simulink model "consolidate_sensors"  (R2025b)
settings: Solver=VariableStepAuto  StartTime=0.0  StopTime=10.0  RelTol=1e-3
settings Model: Creator=atcushen  LastModifiedBy=atcushen

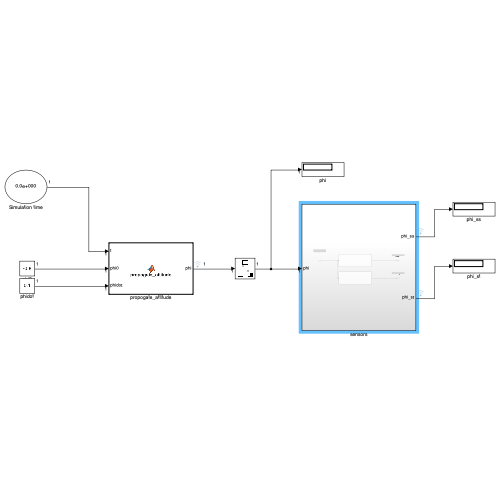
[thumbnail: Simulink's stored preview of the top-level diagram]
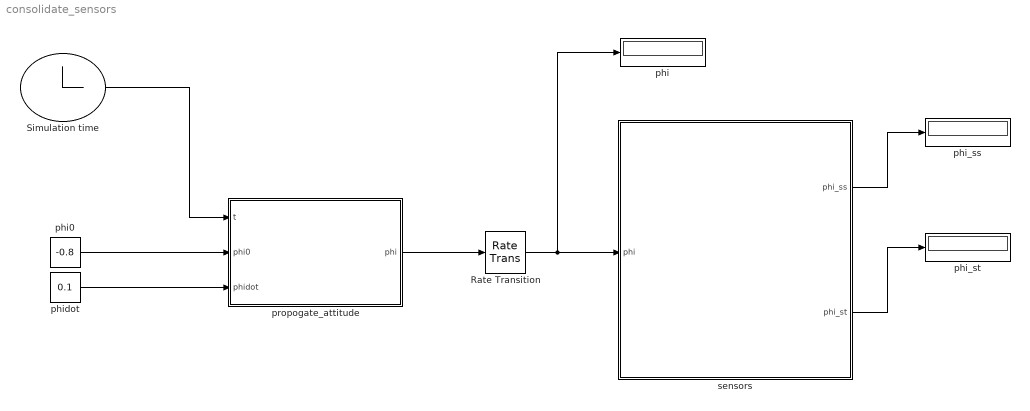
== system consolidate_sensors ==
  Rate Transition : RateTransition  OutPortSampleTime=0.5
  Simulation time : Clock
  phi : Display
  phi0 : Constant  Value=-0.8
  phi_ss : Display
  phi_st : Display
  phidot : Constant  Value=0.1
  propogate_attitude : MATLAB Function  TreatAsAtomicUnit=on
  sensors : Subsystem
  wires:
  sensors/2(phi_st) -> phi_st/1
  Rate Transition/1 -> phi/1, sensors/1(phi)
  phidot/1 -> propogate_attitude/3(phidot)
  Simulation time/1 -> propogate_attitude/1(t)
  phi0/1 -> propogate_attitude/2(phi0)
  sensors/1(phi_ss) -> phi_ss/1
  propogate_attitude/1(phi) -> Rate Transition/1

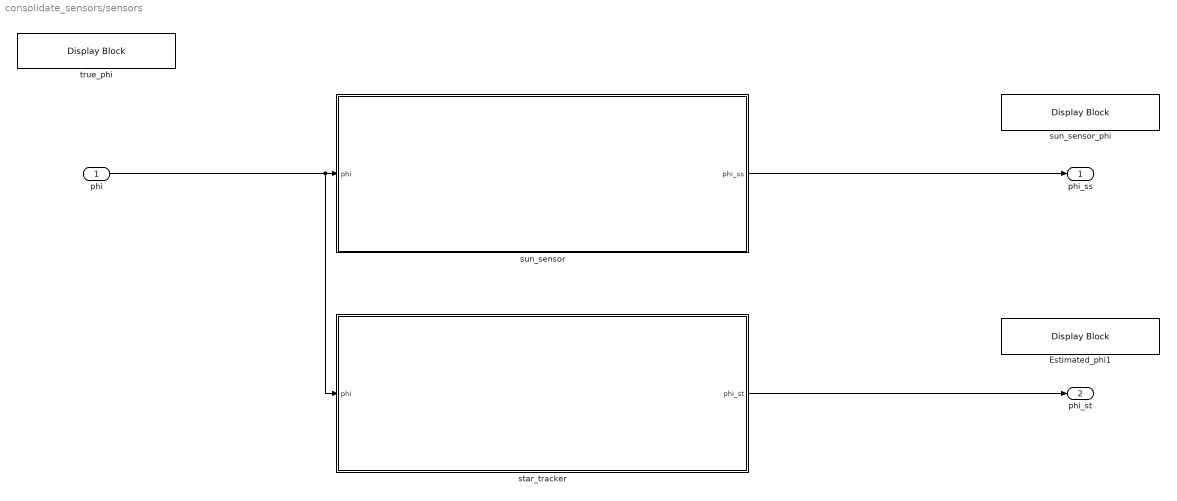
== system consolidate_sensors/sensors ==
  phi : Inport
  Estimated_phi1 : DisplayBlock  LabelPosition=Bottom  Transparency=1  GridColor=[0.502, 0.502, 0.502]
  star_tracker : Subsystem
  sun_sensor : Subsystem
  sun_sensor_phi : DisplayBlock  LabelPosition=Bottom  Transparency=1  GridColor=[0.502, 0.502, 0.502]
  true_phi : DisplayBlock  LabelPosition=Hide  Transparency=1  GridColor=[0.502, 0.502, 0.502]
  phi_ss : Outport
  phi_st : Outport  Port=2
  wires:
  phi/1 -> star_tracker/1(phi), sun_sensor/1(phi)
  sun_sensor/1(phi_ss) -> phi_ss/1
  star_tracker/1(phi_st) -> phi_st/1

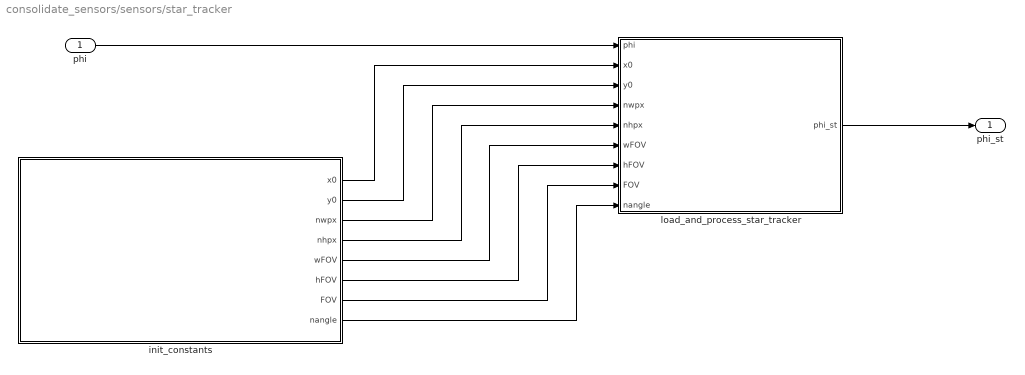
== system consolidate_sensors/sensors/star_tracker ==
  phi : Inport
  init_constants : MATLAB Function  TreatAsAtomicUnit=on
  load_and_process_star_tracker : MATLAB Function  TreatAsAtomicUnit=on
  phi_st : Outport
  wires:
  load_and_process_star_tracker/1(phi_st) -> phi_st/1
  init_constants/1(x0) -> load_and_process_star_tracker/2(x0)
  phi/1 -> load_and_process_star_tracker/1(phi)
  init_constants/2(y0) -> load_and_process_star_tracker/3(y0)
  init_constants/3(nwpx) -> load_and_process_star_tracker/4(nwpx)
  init_constants/4(nhpx) -> load_and_process_star_tracker/5(nhpx)
  init_constants/5(wFOV) -> load_and_process_star_tracker/6(wFOV)
  init_constants/6(hFOV) -> load_and_process_star_tracker/7(hFOV)
  init_constants/7(FOV) -> load_and_process_star_tracker/8(FOV)
  init_constants/8(nangle) -> load_and_process_star_tracker/9(nangle)

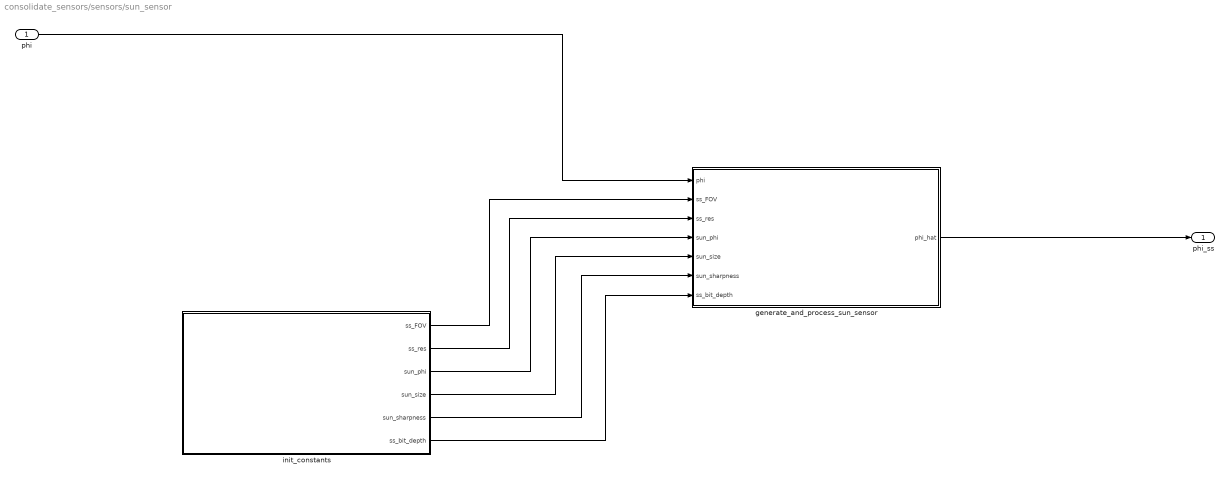
== system consolidate_sensors/sensors/sun_sensor ==
  phi : Inport
  generate_and_process_sun_sensor : MATLAB Function  TreatAsAtomicUnit=on
  init_constants : MATLAB Function  TreatAsAtomicUnit=on
  phi_ss : Outport
  wires:
  phi/1 -> generate_and_process_sun_sensor/1(phi)
  init_constants/5(sun_sharpness) -> generate_and_process_sun_sensor/6(sun_sharpness)
  init_constants/1(ss_FOV) -> generate_and_process_sun_sensor/2(ss_FOV)
  init_constants/2(ss_res) -> generate_and_process_sun_sensor/3(ss_res)
  init_constants/4(sun_size) -> generate_and_process_sun_sensor/5(sun_size)
  init_constants/3(sun_phi) -> generate_and_process_sun_sensor/4(sun_phi)
  init_constants/6(ss_bit_depth) -> generate_and_process_sun_sensor/7(ss_bit_depth)
  generate_and_process_sun_sensor/1(phi_hat) -> phi_ss/1

== matlab function consolidate_sensors/propogate_attitude ==
  data: t input; phi output; phi0 input; phidot input
% propogate attitude
function phi = propogate_attitude(t,phi0,phidot)
    % Input: 
    % t: float, current time, in s
    % phi0: float, initial attitude, in radians
    % phidot: float, rotation rate, in rad/sec
    
    % Output:
    % phi: float, current attitude, in rad/sec

    phi = mod(t*phidot + phi0 + pi,2*pi) - pi;
end

== matlab function consolidate_sensors/sensors/star_tracker/load_and_process_star_tracker ==
  data: phi_st output; phi input; x0 input; y0 input; nwpx input; nhpx input; wFOV input; hFOV input; FOV input; nangle input
function phi_st  = load_and_process_star_tracker(phi,x0,y0,nwpx,nhpx,wFOV,hFOV,FOV,nangle)
    
    % DEFINE PATHS TO STARFIELD IMAGE AND STARTABLE
    starfield_path = 'star_field2.mat'; % str, name of reference photo of full starfield image (which nwpx,wFOV etc describe)
    startable_path = 'star_table2.mat'; % str, name of table which identifies star locations, in radians 


    % PART 1: LOAD STAR TABLE
    
    struct = load(startable_path);
    star_table = struct.star_table;


    % PART 2: GENERATE LOOKUP TABLE

    % Input
    % star_table: nx3 array, from generate_star_table
    % nangle: integer, how many stars to compute angles to from reference
    % star

    % Output
    % star_lookup: nxnagle array, each row corresponds to given row in
    % star_table, columns are angular distances to nangle closest stars

    % Initialize lookup table
    star_lookup = zeros(size(star_table, 1), nangle);

    % Iterate through each star in the table
    for istar = 1:length(star_table)
        
        % Compute the angular distances from the current star to all other stars
        phi_diff = star_table(istar, 1) - star_table(:, 1);
        theta_diff = star_table(istar, 2) - star_table(:, 2);
        angle_diff = sqrt(phi_diff.^2 + theta_diff.^2);

        % Sort the angular distances and get the indices of the smallest values
        [sorted_angles, ~] = sort(angle_diff);
        star_lookup(istar, :) = sorted_angles(2:min(nangle+1, length(sorted_angles))); % Store the smallest values

    
    % PART 3: LOAD STARFIELD REFERENCE IMAGE, AND CROP TO DESIRED FOV

    % Input
    % image: str, path to .png field to import of starfield
    % phi: float, boresight angle of camera, in radians, from -pi to pi
    % FOV: float, angular field of view of camera, in radians, from 0 to 2pi
    % x0: int, x pixel coord of reference star 
    % y0: int, x pixel coord of reference star 
    % nwpx: int, number of pixels of width of starfield image
    % nhpx: int, number of pixels of height of starfield image
    % wFOV: float, field of view width of starfield image [deg]
    % hFOV: float, field of view height of starfield image [deg]
    % Output:
    % st_im: nres x nres array, representing synethic star tracker image

    % Load the .png image as a black and white image array
    file = load(starfield_path);
    img = file.img; 
    starfield_im = rgb2gray(img); % Convert the image to grayscale
    starfield_im = flip(starfield_im,1); % Image array is upside down)

    % Create coordinate axes
    x_ax = 1:nwpx - x0;
    y_ax = 1:nhpx - y0;
    phi_ax = x_ax * pi/180 * wFOV/nwpx;
    theta_ax = y_ax * pi/180 * hFOV/nhpx;
    
    % Crop the starfield image based on the field of view and the phi axis
    phi_indices = phi_ax >= (phi - FOV/2) & phi_ax <= (phi + FOV/2);
    theta_indices = theta_ax >= (-FOV/2) & theta_ax <= (FOV/2); %y0-round(nres/2):y0-round(nres/2)+nres-1;
    
    % Crop the image
    st_im = starfield_im(theta_indices, phi_indices);


    % PART 4: IDENTIFY STAR PIXEL CLUSTERS IN IMAGE

      % Input:
    % st_im: nxn array, representing image from star tracker
    % FOV: float, field of view along each edge of image
    % Output:
    % star_ls: nx2 array, the phi and theta positions (relative to the
    % center of the image) for each star identified
    
    % Get image dimensions (not passed to function call)
    [theta_nres,phi_nres] = size(st_im);
    
    % Convert coordinates to phi and theta positions
    phi_positions = linspace(-FOV/2, FOV/2, phi_nres);
    theta_positions = linspace(-FOV/2, FOV/2, theta_nres);
    
    % Identify bright points in the star tracker image
     threshold = 0.3 * 255; % Set a threshold to identify bright points
    % Create filtered im
     filtered_im = zeros(size(st_im)); % Initialize filtered image
     filtered_im(st_im > threshold) = 1; % Set values to 1 where st_im exceeds threshold
    % Find connected components
     CC = bwconncomp(filtered_im);
    % Create label matrix - CHANGED FOR CODEGEN
     L = zeros(size(filtered_im), 'uint16');
     for k = 1:CC.NumObjects
         L(CC.PixelIdxList{k}) = k;
     end
    % Create output array for star positions
     star_ls = zeros(max(L(:)), 2);
    % Iterate through each connected component
    for jstar = 1:max(L(:))
    % Get the coordinates of the current star cluster
     [y_cluster, x_cluster] = find(L == jstar);
    % Store the average position of the cluster
     star_ls(jstar, 1) = mean(phi_positions(x_cluster)); % Average phi coordinate
     star_ls(jstar, 2) = mean(theta_positions(y_cluster)); % Average theta coordinate
    end

    % PART 5: MATCH IDENTIFIED STARS TO LOOKUP TABLE

    % Input
    % star_ls: nx2 array, the phi and theta positions (relative to the
    % center of the image) for each star identified
    % star_pos_error: float, angular uncertainty in position of stars
    % star_lookup: nxnagle array, each row corresponds to given row in
    % star_table, columns are angular distances to closest stars

    % Output
    % star_num: integer, index number of matched star
    % deltaphi: float, offset in phi of matched star from image center, in radians
    % deltatheta: float, offset in phi of matched star from image center, in radians
    % match_status: integer, 0=failed, 1=matched, 2=multiple matches refined
    % stars_tried: integer, number of stars checked before finding match

    % Compute error bound as single pixel width (radians)
    star_pos_error = wFOV/nwpx * pi/180;

    % CHANGED FOR CODEGEN - Initialize outputs with default values
    star_num = int32(-1);
    deltaphi = 0.0;
    deltatheta = 0.0;
    match_status = int32(0);  % debug output
    stars_tried = int32(0);   % debug output

    % Iterate through stars in image, starting closest to middle, until we
    % get a positive match
    star_match = false;
    
    % Calculate the sum of squares for each star position
    star_ls_dist = sum(star_ls.^2, 2);
    
    % Sort the star_ls based on the sum of squares
    [~, sorted_indices] = sort(star_ls_dist);
    star_ls = star_ls(sorted_indices, :);

    istar = 1;
    while star_match == false && istar <= length(star_ls)
        stars_tried = int32(istar);  % tracking progress
        
        % Compute distances to other stars
        phi_diff = star_ls(istar, 1) - star_ls(:, 1);
        theta_diff = star_ls(istar, 2) - star_ls(:, 2);
        angle_diff = sqrt(phi_diff.^2 + theta_diff.^2);

        % Sort the computed angular distances from smallest to largest
        [sorted_angles, ~] = sort(angle_diff);
        
        % Drop the first element of sorted_angles (distance to itself = 0)
        sorted_angles(1) = [];

        % Reduce sorted angles to only be as long as star_lookup is wide
        sorted_angles = sorted_angles(1:min(length(sorted_angles), size(star_lookup, 2)));

        % Create an array of stars within the positional error range
        match_indices = star_lookup(:, 1) >= (sorted_angles(1) - star_pos_error) & ...
                        star_lookup(:, 1) <= (sorted_angles(1) + star_pos_error);
        matched_stars = star_lookup(match_indices, :);

        % Check if that immediately identified the current state. 
        % If not, compare the angular distances one by one, bringing in more to
        % reduce the number of remaining options
        iangle = 2;

        while size(matched_stars,1) > 1 & iangle <= size(star_lookup,2)
            match_status = int32(2);  % indicates multiple matches being refined
            
            % We loop through the remaining matches
            for j = 1:size(match_indices, 1)
                if j ~= 0
                    % Check to see if the next closest star is within error of
                    % any of the neighbouring stars listed in the lookup table
                    % If none of the angles are close enough, then reject this
                    % match
                    if all(abs(star_lookup(j, iangle:end) - sorted_angles(iangle)) > star_pos_error)
                        match_indices(j) = 0; % Set the jth non-zero element of match_indices to zero
                    end
                end 
            end
            matched_stars = star_lookup(match_indices, :);
        
            iangle = iangle + 1;
        end
        
        % Check if we could use this star 
        if size(matched_stars,1) ~= 1
            % no match found for this star, continue
            istar = istar + 1; % Move to the next star
        else
            % CHANGED FOR CODEGEN - Force scalar by using loop instead of find
            for k = 1:length(match_indices)
                if match_indices(k) ~= 0
                    star_num = int32(k);
                    break;
                end
            end
            deltaphi = star_ls(istar,1); % Offset in phi
            deltatheta = star_ls(istar,2); % Offset in theta
            star_match = true;
            match_status = int32(1);  % successful match
        end
    end

    % Return error if star tracker failed 
    if star_match == false
        % CHANGED FOR CODEGEN - tracker failed
        star_num = int32(-1);
        deltaphi = 0.0;
        deltatheta = 0.0;
        match_status = int32(0);  % Failed to match
    end

    
    % PART 6: COMPUTE PHI_HAT

     % Input
    % star_num: integer, index number of matched star
    % star_table: n_stars x 3 array, where column 1 is phi position of
    % star, column 2 is theta position, column 3 is relative brightness
    % deltaphi: float, offset in phi of matched star from image center, in
    % radians
    
    % Output
    % boresight_phi: float, actual orientation of the center of the cameras
    % FOV [rad]
    
    if star_num == -1
        phi_st = NaN;
    else 
        phi_st = star_table(star_num,1) - deltaphi;
    end
end

== matlab function consolidate_sensors/sensors/sun_sensor/init_constants ==
  data: ss_FOV output; ss_res output; sun_phi output; sun_size output; sun_sharpness output; ss_bit_depth output
% define all our constants
function [ss_FOV,ss_res,sun_phi,sun_size,sun_sharpness,ss_bit_depth] = init_constants
    % Output
    ss_FOV = pi/4;  % float, sun sensor field of field, in radians 
    ss_res = 64; % int, number of pixels on a side of sun sensor image
    sun_phi = 0; % float, position of sun in sky, in radians
    sun_size = pi/128; % float, angular size of sun, in radians
    sun_sharpness = 3; % float, sun sharpness factor (1-5)
    ss_bit_depth = 63; % int, maximum pixel value of sun sensor image
end

== matlab function consolidate_sensors/sensors/star_tracker/init_constants ==
  data: x0 output; y0 output; nwpx output; nhpx output; wFOV output; hFOV output; FOV output; nangle output
% define all our constants
function [x0,y0,nwpx,nhpx,wFOV,hFOV,FOV,nangle] = init_constants
    % Output
    x0 = 3270;  % int, pixel coords of reference star used to set phi=0
    y0 = 1608; % int, pixel coords of reference star used to set theta=0
    nwpx = 4608; % int, pixel width of full starfield image
    nhpx = 2592; % int, pixel height of full starfield image
    wFOV = 102; % float, angular field of view of reference starfield image width, in degrees
    hFOV = 67; % float, angular field of view of reference starfield image height, in degrees
    FOV = pi/6; % float, chosen field of fiew of cropped starfield image, in radians
    nangle = 10; % int, how many angular distances to compute for each star
end

== matlab function consolidate_sensors/sensors/sun_sensor/generate_and_process_sun_sensor ==
  data: phi input; phi_hat output; ss_FOV input; ss_res input; sun_phi input; sun_size input; sun_sharpness input; ss_bit_depth input
% Generate a synthetic sun sensor IR image, based off present attitude phi
function phi_hat = generate_and_process_sun_sensor(phi,ss_FOV,ss_res,sun_phi,sun_size,sun_sharpness,ss_bit_depth)
    
    % PART 1: GENERATE IMAGE
    
    % Input: 
    % phi: float, current pointing angle, in radians
    % ss_FOV: float, viewing angle of sun sensor in radians
    % ss_res: integer, number of pixels on edge of image
    % sun_phi: float, angular position of sun in radians
    % sun_size: float, angular size of sun in radians
    % sun_sharpness: float, degree of function describing sun shape (higher
    % is sharper), recommended 1-5
    % ss_bit_depth: integer, max brightness value of each pixel
    
    % Output:
    % ss_im: ss_res x ss_res array representing synthetic sun sensor image

    phi_ax = linspace(phi-ss_FOV/2,phi+ss_FOV/2,ss_res); % Determine phi axis of image
    theta_ax = linspace(-ss_FOV/2,ss_FOV/2,ss_res); % Determine theta axis of image

    [phi_im, theta_im] = meshgrid(phi_ax, theta_ax); % Create 2D array of angle coordinates
    
    % Add the sun to the image
    ss_im = ss_bit_depth * exp(-((((phi_im-sun_phi).^2+theta_im.^2)/sun_size^2).^sun_sharpness));

    % Add random noise to the image 
    noise_level = ss_bit_depth*0.05; % Adjust the noise level as needed
    noise = noise_level * randn([ss_res,ss_res]); % Generate Gaussian noise
    ss_im = ss_im + noise; % Add noise to the image
    ss_im(ss_im < 0) = 0; % Ensure no negative value

    % PART 2: PROCESS

    % Input: 
    % ss_im: ss_res x ss_res array representing synthetic sun sensor image
    % ss_FOV: float, viewing angle of sun sensor in radians (assumed
    % square)
    % sun_phi: float, absolute angular position of sun in sky, in radians
    % ss_bit_depth: integer, max brightness value of each pixel
    
    % Output: 
    % phi_hat: float, estimate for current attitude, in radians
    
    % Set threshold; cells dimmer than this will be assumed to not be the
    % sun
    cutoff_brightness = 0.05 * ss_bit_depth;
    
    % Get dimensions of the image
    [~,ss_res] = size(ss_im);
    
    % Sum ss_im along columns to get the total pixel brightness in each column
    col_brightness = sum(ss_im, 1); % Sum along rows to get a 1D array

    % Filter out false negatives
    col_brightness(col_brightness < ss_res * cutoff_brightness) = 0;
     
    % Check for adjacent entries in col_brightness greater than zero
    adjacent_found = false;
    multiple_adjacents = false;
    for i = 1:length(col_brightness)-1
        if col_brightness(i) > 0 && col_brightness(i+1) > 0
            if adjacent_found && col_brightness(i-1) == 0
                multiple_adjacents = true;
            else
                adjacent_found = true;
            end
        end
    end
    
    % Display errors
    if ~adjacent_found 
        disp('ERROR: No sun found in frame');
        phi_hat = NaN; % Return NaN if no adjacent entries are found
        return; % Exit the function early
    elseif multiple_adjacents
        disp('ERROR: Multiple sun-like clusters found, cannot identify the sun');
        phi_hat = NaN; % Return NaN if multiple adjacent entries are found
        return; % Exit the function early
    end
    
    % Iterate over the indices of col_brightness that are greater than zero
    sun_indices = find(col_brightness > 0);
       
    % Get the brightness-weighted pixel location of the sun
    sun_pixel_loc = sum(col_brightness(sun_indices) .* sun_indices) / sum(col_brightness(sun_indices));

    % Determine phi_hat from this relative position
    phi_hat = sun_phi - ((sun_pixel_loc / ss_res) * ss_FOV - ss_FOV/2); % Estimate current attitude
   
end
